simulink model "SM_3_x_Vm_Gsm"  (R2021b)
settings: Solver=VariableStepAuto  StartTime=0.0  StopTime=5  RelTol=1e-3
settings Model: Creator=sama1402  LastModifiedBy=sama1402

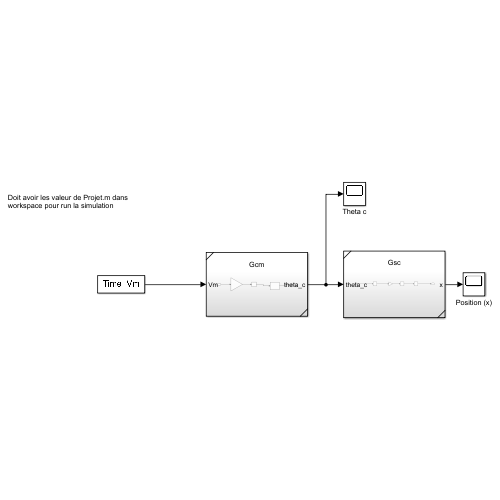
[thumbnail: Simulink's stored preview of the top-level diagram]
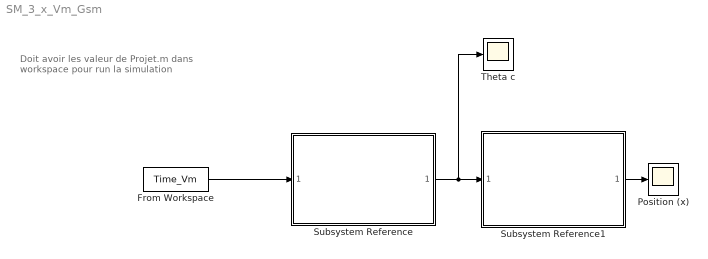
== system SM_3_x_Vm_Gsm ==
  note: Doit avoir les valeur de Projet.m dans workspace pour run la simulation
  From Workspace : FromWorkspace  VariableName=Time_Vm
  Position (x) : Scope
  Subsystem Reference : Subsystem  ReferencedSubsystem=Gcm
  Subsystem Reference1 : Subsystem  ReferencedSubsystem=Gsc
  Theta c : Scope
  wires:
  Subsystem Reference/1 -> Theta c/1, Subsystem Reference1/1
  From Workspace/1 -> Subsystem Reference/1
  Subsystem Reference1/1 -> Position (x)/1
